simulink model "quad_6DOF_quaternion_PD"  (R2023a)
settings: Solver=ode1  StartTime=0.0  StopTime=30  FixedStep=0.01  RelTol=1e-3
libraries: aerolibutil x2, sharedtransform x2, matrix_library x1, simulink_extras x1, sharedutil x1, uavutilslib x1
settings Model: Creator=adan  LastModifiedBy=adan

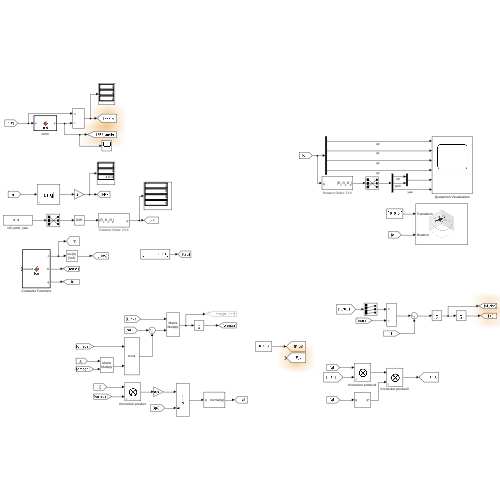
[thumbnail: Simulink's stored preview of the top-level diagram]
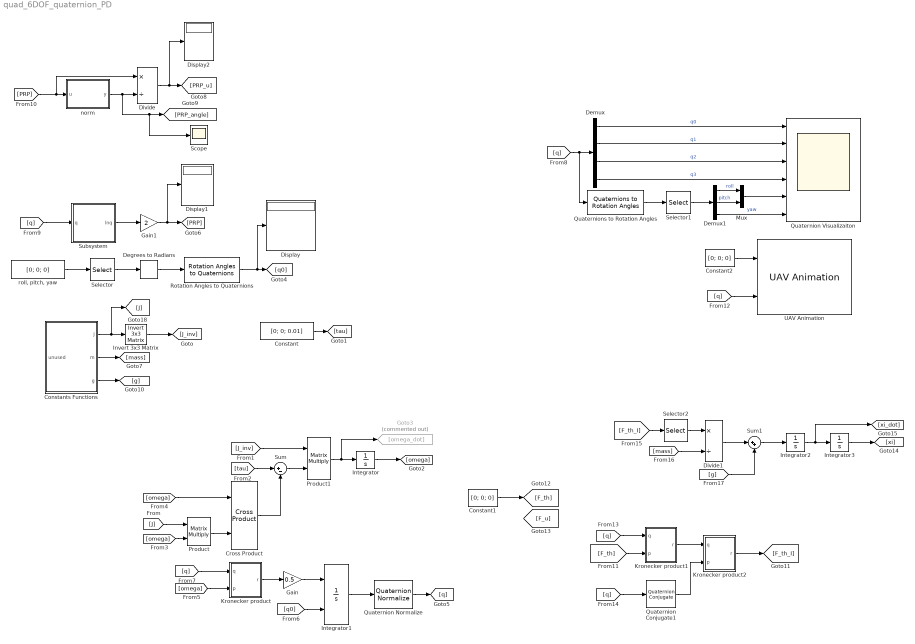
== system quad_6DOF_quaternion_PD ==
  Constant : Constant  Value=[0; 0; 0.01]
  Constant1 : Constant  Value=[0; 0; 0]
  Constant2 : Constant  Value=[0; 0; 0]
  Constants Functions : MATLAB Function  TreatAsAtomicUnit=on
  Cross Product : matrix_library/Cross Product
  Degrees to Radians : simulink_extras/Transformations/Degrees to Radians
  Demux : Demux
  Demux1 : Demux  Outputs=3
  Display : Display
  Display1 : Display
  Display2 : Display
  Divide : Product  Inputs=*/
  Divide1 : Product  Inputs=*/
  Gain : Gain  Gain=0.5
  Gain1 : Gain  Gain=2
  Goto3 : Goto  Commented=on  GotoTag=omega_dot
  Integrator : Integrator  InitialCondition=[0; 0; 0]
  Integrator1 : Integrator  InitialConditionSource=external
  Integrator2 : Integrator  InitialCondition=[0; 0; 0]
  Integrator3 : Integrator  InitialCondition=[0; 0; 0]
  Invert 3x3 Matrix : aerolibutil/Invert  3x3 Matrix
  Kronecker product : Subsystem
  Kronecker product1 : Subsystem
  Kronecker product2 : Subsystem
  Mux : Mux  Inputs=2
  Product : Product  Multiplication=Matrix(*)
  Product1 : Product  Multiplication=Matrix(*)
  Quaternion Conjugate1 : aerolibutil/Quaternion Conjugate
  Quaternion Normalize : sharedutil/Quaternion Normalize  aMode=aMode
  Quaternion Visualizaiton : Scope  NumInputPorts=6
  Quaternions to Rotation Angles : sharedtransform/Quaternions to Rotation Angles  rotationOrder=ZYX  aMode=aMode
  Rotation Angles to Quaternions : sharedtransform/Rotation Angles to Quaternions  rotationOrder=ZYX  aMode=aMode
  Scope : Scope
  Selector : Selector  InputPortWidth=3  IndexOptions=Index vector (dialog)  Indices=[3 2 1]  OutputSizes=1
  Selector1 : Selector  InputPortWidth=3  IndexOptions=Index vector (dialog)  Indices=[3 2 1]  OutputSizes=1
  Selector2 : Selector  InputPortWidth=4  IndexOptions=Index vector (dialog)  Indices=[2:4]  OutputSizes=1
  Subsystem : Subsystem
  Sum : Sum  Inputs=|+-
  Sum1 : Sum  Inputs=|++
  UAV Animation : uavutilslib/UAV Animation  UAVType=Multirotor  UAVSize=1  InertialZDirection=Down  SampleTime=-1
  norm : MATLAB Function  TreatAsAtomicUnit=on
  "roll, pitch, yaw" : Constant  Value=[0; 0; 0]
  wires:
  Constants Functions/1(J) -> [J], Invert 3x3 Matrix/1
  Invert 3x3 Matrix/1 -> [J_inv]
  Constant/1 -> [tau]
  [tau] -> Sum/1
  [J] -> Product/1
  [omega] -> Product/2
  [omega] -> Cross Product/1
  Product/1 -> Cross Product/2
  Cross Product/1 -> Sum/2
  Sum/1 -> Product1/2
  [J_inv] -> Product1/1
  Product1/1 -> Goto3/1, Integrator/1
  Integrator/1 -> [omega]
  [omega] -> Kronecker product/2(p)
  Kronecker product/1(r) -> Gain/1
  Gain/1 -> Integrator1/1
  Degrees to Radians/1 -> Rotation Angles to Quaternions/1
  Selector/1 -> Degrees to Radians/1
  "roll, pitch, yaw"/1 -> Selector/1
  Rotation Angles to Quaternions/1 -> Display/1, [q0]
  [q0] -> Integrator1/2
  Integrator1/1 -> Quaternion Normalize/1
  [q] -> Kronecker product/1(q)
  [q] -> Quaternions to Rotation Angles/1, Demux/1
  Demux/1 -> Quaternion Visualizaiton/1  "q0"
  Demux/2 -> Quaternion Visualizaiton/2  "q1"
  Demux/3 -> Quaternion Visualizaiton/3  "q2"
  Demux/4 -> Quaternion Visualizaiton/4  "q3"
  Quaternions to Rotation Angles/1 -> Selector1/1
  Selector1/1 -> Demux1/1
  Demux1/1 -> Mux/1  "roll"
  Demux1/2 -> Mux/2  "pitch"
  Mux/1 -> Quaternion Visualizaiton/5
  Demux1/3 -> Quaternion Visualizaiton/6  "yaw"
  Quaternion Normalize/1 -> [q]
  [q] -> UAV Animation/2
  Constant2/1 -> UAV Animation/1
  Constants Functions/2(m) -> [mass]
  [q] -> Subsystem/1(q)
  Subsystem/1(lnq) -> Gain1/1
  Gain1/1 -> Display1/1, [PRP]
  [PRP] -> norm/1(u), Divide/1
  norm/1(y) -> Scope/1, [PRP_angle], Divide/2
  Divide/1 -> [PRP_u], Display2/1
  Constants Functions/3(g) -> [g]
  [q] -> Kronecker product1/1(q)
  [F_th] -> Kronecker product1/2(p)
  Kronecker product1/1(r) -> Kronecker product2/1(q)
  Quaternion Conjugate1/1 -> Kronecker product2/2(p)
  [q] -> Quaternion Conjugate1/1
  Kronecker product2/1(r) -> [F_th_I]
  Constant1/1 -> [F_th]
  [F_th_I] -> Selector2/1
  [mass] -> Divide1/2
  Divide1/1 -> Sum1/1
  [g] -> Sum1/2
  Sum1/1 -> Integrator2/1
  Integrator2/1 -> [xi_dot], Integrator3/1
  Integrator3/1 -> [xi]
  Selector2/1 -> Divide1/1

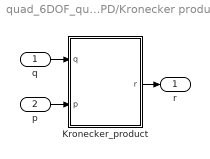
== system quad_6DOF_quaternion_PD/Kronecker product ==
  q : Inport
  p : Inport  Port=2
  Kronecker_product : MATLAB Function  TreatAsAtomicUnit=on
  r : Outport
  wires:
  q/1 -> Kronecker_product/1(q)
  p/1 -> Kronecker_product/2(p)
  Kronecker_product/1(r) -> r/1

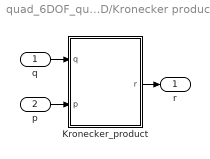
== system quad_6DOF_quaternion_PD/Kronecker product1 ==
  q : Inport
  p : Inport  Port=2
  Kronecker_product : MATLAB Function  TreatAsAtomicUnit=on
  r : Outport
  wires:
  q/1 -> Kronecker_product/1(q)
  p/1 -> Kronecker_product/2(p)
  Kronecker_product/1(r) -> r/1

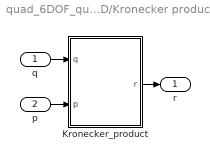
== system quad_6DOF_quaternion_PD/Kronecker product2 ==
  q : Inport
  p : Inport  Port=2
  Kronecker_product : MATLAB Function  TreatAsAtomicUnit=on
  r : Outport
  wires:
  q/1 -> Kronecker_product/1(q)
  p/1 -> Kronecker_product/2(p)
  Kronecker_product/1(r) -> r/1

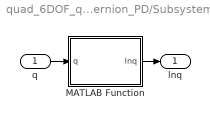
== system quad_6DOF_quaternion_PD/Subsystem ==
  q : Inport
  MATLAB Function : MATLAB Function  TreatAsAtomicUnit=on
  lnq : Outport
  wires:
  MATLAB Function/1(lnq) -> lnq/1
  q/1 -> MATLAB Function/1(q)

== matlab function quad_6DOF_quaternion_PD/Subsystem/MATLAB Function ==
  data: q input; lnq output
function lnq = fcn(q)

if length(q) == 4
    q0 = q(1);
    
    q_vec = [q(2); q(3); q(4)];

    if norm(q_vec) == 0
        lnq = [0; 0; 0];
    else
        lnq = (q_vec / (norm(q_vec)) ) * acos(q0);
    end
else
    error('Input must be a vector 4 by 1 (Quaternion)')
end

== matlab function quad_6DOF_quaternion_PD/Kronecker product/Kronecker_product ==
  data: q input; r output; p input
function r = fcn(q, p)

%{
    Function to describe in matrix math the Kronecker product between
    two quaternions
    
    r = p kronecker q
    %}

    len = length(p);

    if len == 3
        p1 = [0; p];
        q0 = q(1);
        q1 = q(2);
        q2 = q(3);
        q3 = q(4);
        
        % skew symmetric matrix
        q_matrix = [q0, -q1, -q2, -q3;
                  q1, q0, -q3, q2;
                  q2, q3, q0, -q1;
                  q3, -q2, q1, q0];
        
        r = q_matrix * p1;

    elseif len == 4
        q0 = q(1);
        q1 = q(2);
        q2 = q(3);
        q3 = q(4);
        
        % skew symmetric matrix
        q_matrix = [q0, -q1, -q2, -q3;
                  q1, q0, -q3, q2;
                  q2, q3, q0, -q1;
                  q3, -q2, q1, q0];
        
        r = q_matrix * p;

    else
        error('Quaternions dimensions do not match')
    end

== matlab function quad_6DOF_quaternion_PD/Constants Functions ==
  data: unused input; J output; m output; g output
function [J, m, g] = fcn(~)

m = 2.0; % kg

Jxx =  0.0411; % kg m²
Jyy = 0.0478; % kg m²
Jzz = 0.0599; % kg m²

J = [Jxx, 0, 0;
     0, Jyy, 0;
     0, 0, Jzz];

g = [0; 0; 9.81];

== matlab function quad_6DOF_quaternion_PD/norm ==
  data: u input; y output
function y = fcn(u)

y = norm(u);

== matlab function quad_6DOF_quaternion_PD/Kronecker product1/Kronecker_product ==
  data: q input; r output; p input
function r = fcn(q, p)

%{
    Function to describe in matrix math the Kronecker product between
    two quaternions
    
    r = p kronecker q
    %}

    len = length(p);

    if len == 3
        p1 = [0; p];
        q0 = q(1);
        q1 = q(2);
        q2 = q(3);
        q3 = q(4);
        
        % skew symmetric matrix
        q_matrix = [q0, -q1, -q2, -q3;
                  q1, q0, -q3, q2;
                  q2, q3, q0, -q1;
                  q3, -q2, q1, q0];
        
        r = q_matrix * p1;

    elseif len == 4
        q0 = q(1);
        q1 = q(2);
        q2 = q(3);
        q3 = q(4);
        
        % skew symmetric matrix
        q_matrix = [q0, -q1, -q2, -q3;
                  q1, q0, -q3, q2;
                  q2, q3, q0, -q1;
                  q3, -q2, q1, q0];
        
        r = q_matrix * p;

    else
        error('Quaternions dimensions do not match')
    end

== matlab function quad_6DOF_quaternion_PD/Kronecker product2/Kronecker_product ==
  data: q input; r output; p input
function r = fcn(q, p)

%{
    Function to describe in matrix math the Kronecker product between
    two quaternions
    
    r = p kronecker q
    %}

    len = length(p);

    if len == 3
        p1 = [0; p];
        q0 = q(1);
        q1 = q(2);
        q2 = q(3);
        q3 = q(4);
        
        % skew symmetric matrix
        q_matrix = [q0, -q1, -q2, -q3;
                  q1, q0, -q3, q2;
                  q2, q3, q0, -q1;
                  q3, -q2, q1, q0];
        
        r = q_matrix * p1;

    elseif len == 4
        q0 = q(1);
        q1 = q(2);
        q2 = q(3);
        q3 = q(4);
        
        % skew symmetric matrix
        q_matrix = [q0, -q1, -q2, -q3;
                  q1, q0, -q3, q2;
                  q2, q3, q0, -q1;
                  q3, -q2, q1, q0];
        
        r = q_matrix * p;

    else
        error('Quaternions dimensions do not match')
    end
